simulink model "speed_verification_System"  (R2024a)
settings: Solver=VariableStepAuto  StartTime=0.0  StopTime=10.0  RelTol=1e-3
libraries: simulink x4
settings Model: Creator=admin  LastModifiedBy=admin

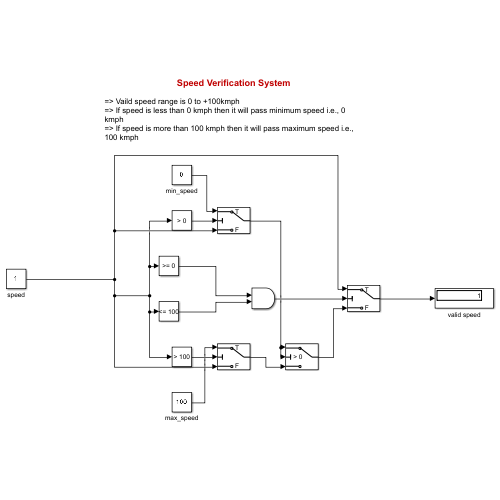
[thumbnail: Simulink's stored preview of the top-level diagram]
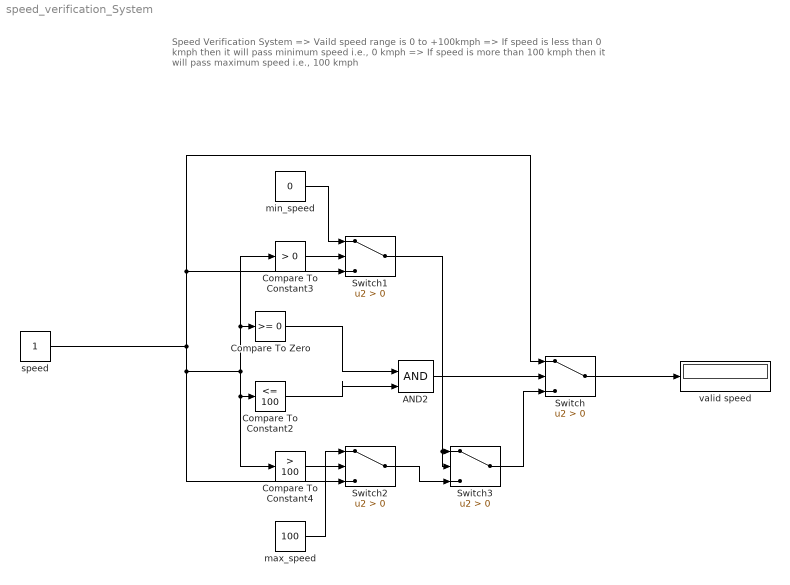
== system speed_verification_System ==
  note: Speed Verification System
      |
      | => Vaild speed range is 0 to +100kmph
      | => If speed is less than 0 kmph then it will pass minimum speed i.e., 0 kmph
      | => If speed is more than 100 kmph then it will pass maximum speed i.e., 100 kmph
  AND2 : Logic  IconShape=distinctive  AllPortsSameDT=off  OutDataTypeStr=boolean
  Compare To Constant2 : simulink/Logic and Bit Operations/Compare To Constant  relop=<=  const=100  OutDataTypeStr=boolean
  Compare To Constant3 : simulink/Logic and Bit Operations/Compare To Constant  relop=>  const=0  OutDataTypeStr=boolean
  Compare To Constant4 : simulink/Logic and Bit Operations/Compare To Constant  relop=>  const=100  OutDataTypeStr=boolean
  Compare To Zero : simulink/Logic and Bit Operations/Compare To Zero  relop=>=  OutDataTypeStr=boolean
  Switch{,1..3} (4 alike) : Switch  Criteria=u2 > Threshold  SaturateOnIntegerOverflow=off  InputSameDT=off
  max_speed : Constant  Value=100
  min_speed : Constant  Value=0
  speed : Constant
  valid speed : Display
  wires:
  Switch/1 -> valid speed/1
  Switch3/1 -> Switch/3
  Compare To Constant2/1 -> AND2/2
  Compare To Zero/1 -> AND2/1
  AND2/1 -> Switch/2
  Compare To Constant4/1 -> Switch2/2
  Compare To Constant3/1 -> Switch1/2
  max_speed/1 -> Switch2/1
  min_speed/1 -> Switch1/1
  Switch2/1 -> Switch3/3
  speed/1 -> Switch2/3, Compare To Constant3/1, Compare To Zero/1, Compare To Constant4/1, Compare To Constant2/1, Switch/1, Switch1/3
  Switch1/1 -> Switch3/1, Switch3/2
